simulink model "model"  (R2014a)
settings: Solver=FixedStepDiscrete  StartTime=0.0  StopTime=10  RelTol=1e-3
values from neighbouring files (symbols this model uses):
  BufLen = 4*Fs    [init_model.m]
  delay_fp1 = ceil(delay_qrs-fpdl-fpdi-fpdd)    [init_model.m]
  delay_fp2 = ceil(delay_qrs-fpdl-s)    [init_model.m]
  delay_noise = ceil(noiseds + noisedl)    [init_model.m]
  Fs = signal.fs    [init_model.m]
  s = round(0.06*Fs)    [init_model.m]
undefined symbols (not defined in the file or in its folder): fpad, fpai, fpal, fpbd, fpbi, fpbl, FrameLen, get, gopalakhermite, HR, JayMeasurePts, noiseal, noiseas, noisebl, noisebs, qrsad, qrsah, qrsai, qrsal, qrsbd, qrsbh, qrsbi, qrsbl, qrsgh, qrsgl, rochahermite1, rochahermite2, stlen
undefined symbols (not defined in the file): L1, L2, L3, L4, newL1, newL2
libraries: simulink x16, neural x14, dspbuff3 x4, dspsigops x2, dspsnks4 x1
(part 1 of 2)
Description:
  | Real-time simulation of ECG ischemia detection
settings Model: Creator=Diego Sogari  LastModifiedBy=Usuario

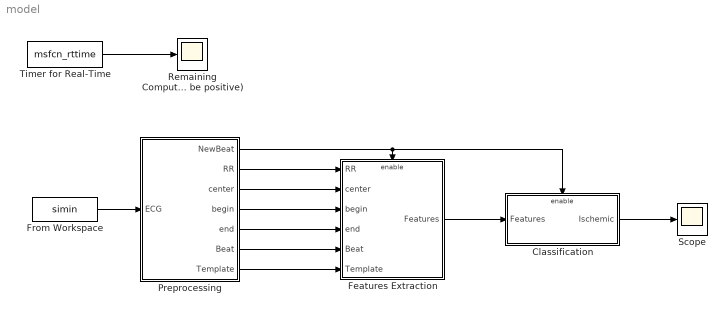
== system model ==
  Classification : Subsystem
  Features Extraction : Subsystem
  From Workspace : FromWorkspace  VariableName=simin  SampleTime=1/Fs  Interpolate=off  OutputAfterFinalValue=Setting to zero
  Preprocessing : Subsystem
  Remaining Computation Time (must be positive) : Scope
      settings: TimeRange=10  YMin=-0.175  YMax=0.025
  Scope : Scope
  Timer for Real-Time : S-Function  FunctionName=msfcn_rttime  Parameters=Fs 1  EnableBusSupport=off
  wires:
  From Workspace/1 -> Preprocessing/1(ECG)
  Preprocessing/5(end) -> Features Extraction/4(end)
  Preprocessing/2(RR) -> Features Extraction/1(RR)
  Preprocessing/3(center) -> Features Extraction/2(center)
  Preprocessing/4(begin) -> Features Extraction/3(begin)
  Classification/1(Ischemic) -> Scope/1
  Timer for Real-Time/1 -> Remaining Computation Time (must be positive)/1
  Preprocessing/1(NewBeat) -> Classification/Enable, Features Extraction/Enable
  Preprocessing/6(Beat) -> Features Extraction/5(Beat)
  Preprocessing/7(Template) -> Features Extraction/6(Template)
  Features Extraction/1(Features) -> Classification/1(Features)

== system model/Classification ==
  Features : Inport
  Enable : EnablePort
  Bus Selector : BusSelector
  Gopalak Networks : Subsystem
  Mohebbi Netowrk : Subsystem
  Rocha Networks : Subsystem
  Vector Concatenate : Concatenate  NumInputs=3
  Ischemic : Outport
  wires:
  Features/1 -> Bus Selector/1
  Bus Selector/3 -> Gopalak Networks/1(Features)  "<signal3>"
  Bus Selector/1 -> Rocha Networks/1(Features)  "<signal1>"
  Bus Selector/2 -> Mohebbi Netowrk/1(Features)  "<signal2>"
  Rocha Networks/1(Ischemic) -> Vector Concatenate/1
  Mohebbi Netowrk/1(Ischemic) -> Vector Concatenate/2
  Gopalak Networks/1(Ischemic) -> Vector Concatenate/3
  Vector Concatenate/1 -> Ischemic/1

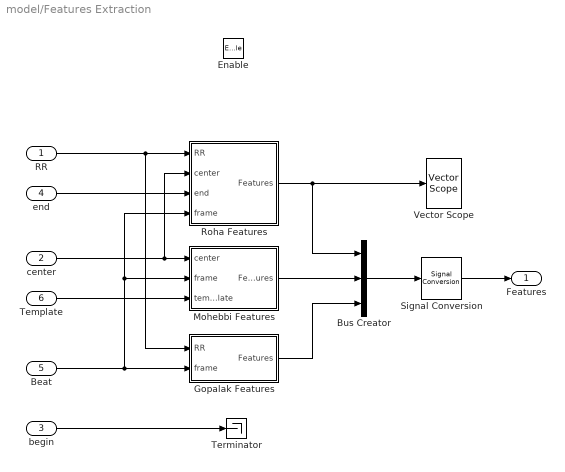
== system model/Features Extraction ==
  RR : Inport
  center : Inport  Port=2
  begin : Inport  Port=3
  end : Inport  Port=4
  Beat : Inport  Port=5
  Template : Inport  Port=6
  Enable : EnablePort
  Bus Creator : BusCreator  Inputs=3
  Gopalak Features : Subsystem
  Mohebbi Features : Subsystem
  Roha Features : Subsystem
  Signal Conversion : SignalConversion
  Terminator : Terminator
  Vector Scope : dspsnks4/Vector Scope  ScopeProperties=on  Domain=Time  HorizSpan=1  DisplayProperties=off  AxisGrid=on  Memory=off  FrameNumber=on  AxisLegend=off  AxisZoom=off  OpenScopeAtSimStart=on  OpenScopeImmediately=off  FigPos=get(0,'defaultfigureposition')  AxisProperties=off  XUnits=Hertz  XRange=[0...Fs/2]  InheritXIncr=on  XIncr=1  XLabel=Time  XLimit=Auto  XMin=0  XMax=1  XStart=0  YUnits=dB  YLabel=Amplitude  LineProperties=off  XAxisParamsVer=6.9
      settings: YMin=-10  YMax=10
  Features : Outport
  wires:
  center/1 -> Roha Features/2(center), Mohebbi Features/1(center)
  RR/1 -> Gopalak Features/1(RR), Roha Features/1(RR)
  end/1 -> Roha Features/3(end)
  Mohebbi Features/1(Features) -> Bus Creator/2
  Roha Features/1(Features) -> Vector Scope/1, Bus Creator/1
  Gopalak Features/1(Features) -> Bus Creator/3
  Beat/1 -> Roha Features/4(frame), Mohebbi Features/2(frame), Gopalak Features/2(frame)
  Template/1 -> Mohebbi Features/3(template)
  begin/1 -> Terminator/1
  Bus Creator/1 -> Signal Conversion/1
  Signal Conversion/1 -> Features/1

== system model/Preprocessing ==
  ECG : Inport
  Filtering : Subsystem
  Subsystem : Subsystem
  NewBeat : Outport
  RR : Outport  Port=2
  center : Outport  Port=3
  begin : Outport  Port=4
  end : Outport  Port=5
  Beat : Outport  Port=6
  Template : Outport  Port=7
  wires:
  ECG/1 -> Filtering/1(Data)
  Filtering/1(QRSsig) -> Subsystem/1(QRSsig)
  Filtering/2(FPsigD) -> Subsystem/2(FPsigD)
  Filtering/3(FPsigM) -> Subsystem/3(FPsigM)
  Filtering/4(Noissig) -> Subsystem/4(Noissig)
  Subsystem/2(RR) -> RR/1
  Subsystem/3(center) -> center/1
  Subsystem/4(begin) -> begin/1
  Subsystem/5(end) -> end/1
  Subsystem/1(NewBeat) -> NewBeat/1
  Subsystem/7(Template) -> Template/1
  Subsystem/6(Beat) -> Beat/1

== system model/Classification/Gopalak Networks ==
  Features : Inport
  Constant : Constant  Value=0  OutDataTypeStr=boolean
  Terminator : Terminator
  Ischemic : Outport
  wires:
  Features/1 -> Terminator/1
  Constant/1 -> Ischemic/1

== system model/Classification/Mohebbi Netowrk ==
  Features : Inport
  Constant : Constant  Value=0  OutDataTypeStr=boolean
  Terminator : Terminator
  Ischemic : Outport
  wires:
  Features/1 -> Terminator/1
  Constant/1 -> Ischemic/1

== system model/Classification/Rocha Networks ==
  Features : Inport
  Compare To Zero : simulink/Logic and Bit Operations/Compare To Zero  relop=>  OutDataTypeStr=boolean
  Feed-Forward Neural Network : Subsystem
      mask help: Feed-Forward Neural Network
      mask Display: e = 0.06;c1 = [120 150 230]/255;c2 = ([120 150 230]+0)/383;c3 = ([120 150 230]+128)/383;patch([0 1 1 0],[0 0 1 1],c1);patch([0 1 1 1-e 1-e 0+e],[0 0 1 1-e 0+e 0+e],c2);patch([0 0 1 1-e 0+e 0+e],[0 1 1 1-e 1-e 0+e],c3);plot([0 1 1 0 0],[0 0 1 1 0]);fprintf('NNET');port_label('input',1,' Input');port_label('output',1,'Output ');
  Ischemic : Outport
  wires:
  Features/1 -> Feed-Forward Neural Network/1(Input)
  Feed-Forward Neural Network/1(Output) -> Compare To Zero/1
  Compare To Zero/1 -> Ischemic/1

== system model/Features Extraction/Gopalak Features ==
  RR : Inport
  frame : Inport  Port=2
  Constant : Constant  Value=gopalakhermite
  Extract Segment : S-Function  FunctionName=msfcn_segmentextractor  Parameters=Fs gopalaksegsize resamplen  EnableBusSupport=off
  Matrix Multiply : Product  Multiplication=Matrix(*)
  segment limits : Subsystem
  Features : Outport
  wires:
  frame/1 -> Extract Segment/1
  RR/1 -> segment limits/1(RR)
  segment limits/1(start) -> Extract Segment/2
  segment limits/2(end) -> Extract Segment/3
  Extract Segment/1 -> Matrix Multiply/2
  Matrix Multiply/1 -> Features/1
  Constant/1 -> Matrix Multiply/1

== system model/Features Extraction/Mohebbi Features ==
  center : Inport
  frame : Inport  Port=2
  template : Inport  Port=3
  Extract ST segment : Subsystem
  Exttract ST difference : Subsystem
  Flsg : Subsystem  mask{trigg=3}
      mask prompts: trigg "Trigger count"
  Sample and Hold : dspsigops/Sample and Hold  trig=Rising edge  initCond=0  latchinput=off
  Sample and Hold1 : dspsigops/Sample and Hold  trig=Rising edge  initCond=0  latchinput=off
  Features : Outport
  wires:
  Sample and Hold/1 -> Extract ST segment/1(frame)
  Exttract ST difference/1(STdiff) -> Features/1
  center/1 -> Extract ST segment/2(center), Exttract ST difference/2(center)
  Flsg/1(flag) -> Sample and Hold1/1, Sample and Hold1/Trigger, Sample and Hold/Trigger
  Sample and Hold1/1 -> Exttract ST difference/Enable
  frame/1 -> Exttract ST difference/3(frame)
  template/1 -> Sample and Hold/1
  Extract ST segment/1(STseg) -> Exttract ST difference/1(refST)

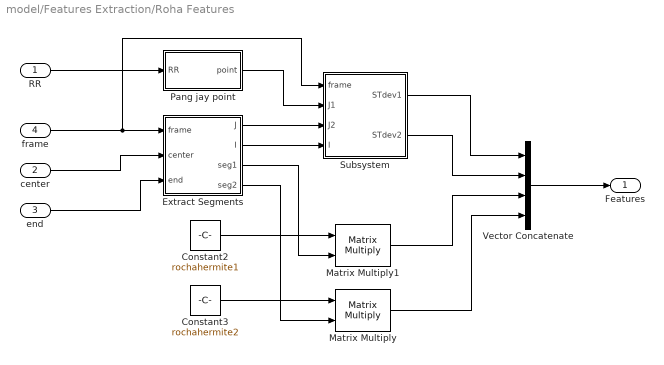
== system model/Features Extraction/Roha Features ==
  RR : Inport
  center : Inport  Port=2
  end : Inport  Port=3
  frame : Inport  Port=4
  Constant2 : Constant  Value=rochahermite1
  Constant3 : Constant  Value=rochahermite2
  Extract Segments : Subsystem
  Matrix Multiply : Product  Multiplication=Matrix(*)
  Matrix Multiply1 : Product  Multiplication=Matrix(*)
  Pang jay point : Subsystem
  Subsystem : Subsystem
  Vector Concatenate : Concatenate  NumInputs=4
  Features : Outport
  wires:
  RR/1 -> Pang jay point/1(RR)
  frame/1 -> Extract Segments/1(frame), Subsystem/1(frame)
  center/1 -> Extract Segments/2(center)
  end/1 -> Extract Segments/3(end)
  Constant2/1 -> Matrix Multiply1/1
  Extract Segments/4(seg2) -> Matrix Multiply/2
  Extract Segments/3(seg1) -> Matrix Multiply1/2
  Matrix Multiply1/1 -> Vector Concatenate/3
  Matrix Multiply/1 -> Vector Concatenate/4
  Vector Concatenate/1 -> Features/1
  Constant3/1 -> Matrix Multiply/1
  Pang jay point/1(point) -> Subsystem/2(J1)
  Extract Segments/1(J) -> Subsystem/3(J2)
  Extract Segments/2(I) -> Subsystem/4(I)
  Subsystem/1(STdev1) -> Vector Concatenate/1
  Subsystem/2(STdev2) -> Vector Concatenate/2

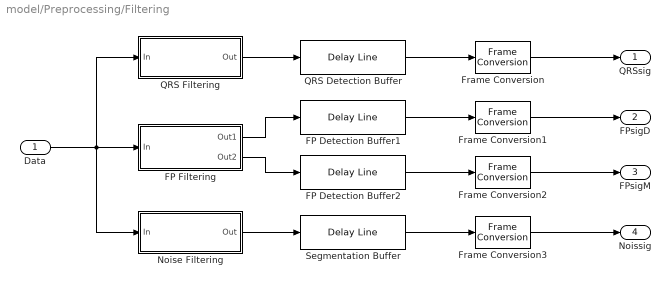
== system model/Preprocessing/Filtering ==
  Data : Inport
  FP Detection Buffer1 : dspbuff3/Delay Line  siz=BufLen  ic=0  directfeed=on  enable_output=off  hold_output=off  TreatMby1Signals=One channel
  FP Detection Buffer2 : dspbuff3/Delay Line  siz=BufLen  ic=0  directfeed=on  enable_output=off  hold_output=off  TreatMby1Signals=One channel
  FP Filtering : Subsystem
  Frame Conversion{,1..3} (4 alike) : FrameConversion  OutFrame=Sample-based
  Noise Filtering : Subsystem
  QRS Detection Buffer : dspbuff3/Delay Line  siz=BufLen  ic=0  directfeed=on  enable_output=off  hold_output=off  TreatMby1Signals=One channel
  QRS Filtering : Subsystem
  Segmentation Buffer : dspbuff3/Delay Line  siz=BufLen  ic=0  directfeed=on  enable_output=off  hold_output=off  TreatMby1Signals=One channel
  QRSsig : Outport
  FPsigD : Outport  Port=2
  FPsigM : Outport  Port=3
  Noissig : Outport  Port=4
  wires:
  Frame Conversion1/1 -> FPsigD/1
  Frame Conversion3/1 -> Noissig/1
  Noise Filtering/1(Out) -> Segmentation Buffer/1
  FP Detection Buffer1/1 -> Frame Conversion1/1
  FP Detection Buffer2/1 -> Frame Conversion2/1
  QRS Filtering/1(Out) -> QRS Detection Buffer/1
  Data/1 -> Noise Filtering/1(In), QRS Filtering/1(In), FP Filtering/1(In)
  FP Filtering/1(Out1) -> FP Detection Buffer1/1
  QRS Detection Buffer/1 -> Frame Conversion/1
  FP Filtering/2(Out2) -> FP Detection Buffer2/1
  Segmentation Buffer/1 -> Frame Conversion3/1
  Frame Conversion2/1 -> FPsigM/1
  Frame Conversion/1 -> QRSsig/1

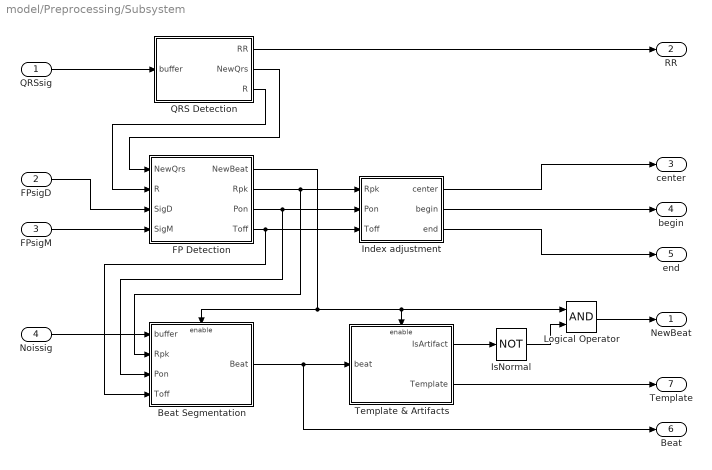
== system model/Preprocessing/Subsystem ==
  QRSsig : Inport
  FPsigD : Inport  Port=2
  FPsigM : Inport  Port=3
  Noissig : Inport  Port=4
  Beat Segmentation : Subsystem
  FP Detection : Subsystem
  Index adjustment : Subsystem
  IsNormal : Logic  Operator=NOT  AllPortsSameDT=off  OutDataTypeStr=boolean
  Logical Operator : Logic  AllPortsSameDT=off  OutDataTypeStr=boolean
  QRS Detection : Subsystem
  Template & Artifacts : Subsystem
  NewBeat : Outport
  RR : Outport  Port=2
  center : Outport  Port=3
  begin : Outport  Port=4
  end : Outport  Port=5
  Beat : Outport  Port=6
  Template : Outport  Port=7
  wires:
  Beat Segmentation/1(Beat) -> Beat/1, Template & Artifacts/1(beat)
  Noissig/1 -> Beat Segmentation/1(buffer)
  FPsigD/1 -> FP Detection/3(SigD)
  QRSsig/1 -> QRS Detection/1(buffer)
  FPsigM/1 -> FP Detection/4(SigM)
  FP Detection/3(Pon) -> Index adjustment/2(Pon), Beat Segmentation/3(Pon)
  QRS Detection/2(NewQrs) -> FP Detection/1(NewQrs)
  QRS Detection/3(R) -> FP Detection/2(R)
  QRS Detection/1(RR) -> RR/1
  FP Detection/2(Rpk) -> Index adjustment/1(Rpk), Beat Segmentation/2(Rpk)
  FP Detection/1(NewBeat) -> Beat Segmentation/Enable, Logical Operator/1, Template & Artifacts/Enable
  Index adjustment/3(end) -> end/1
  FP Detection/4(Toff) -> Index adjustment/3(Toff), Beat Segmentation/4(Toff)
  IsNormal/1 -> Logical Operator/2
  Logical Operator/1 -> NewBeat/1
  Index adjustment/2(begin) -> begin/1
  Template & Artifacts/1(IsArtifact) -> IsNormal/1
  Template & Artifacts/2(Template) -> Template/1
  Index adjustment/1(center) -> center/1

== system model/Classification/Rocha Networks/Feed-Forward Neural Network ==
  Input : Inport  PortDimensions=14  SampleTime=0.004
      mask Display: e = 0.06;c1 = [120 230 180]/255;c2 = ([120 230 180]+0)/(256+128);c3 = ([120 230 180]+128)/(256+128);patch([0 1 1 0],[0 0 1 1],c1);patch([0 1 1 1-e 1-e 0+e],[0 0 1 1-e 0+e 0+e],c2);patch([0 0 1 1-e 0+e 0+e],[0 1 1 1-e 1-e 0+e],c3);plot([0 1 1 0 0],[0 0 1 1 0]);
  Layer 1 : Subsystem
      mask Display: e = 0.06;c1 = [120 150 230]/255;c2 = ([120 150 230]+0)/383;c3 = ([120 150 230]+128)/383;patch([0 1 1 0],[0 0 1 1],c1);patch([0 1 1 1-e 1-e 0+e],[0 0 1 1-e 0+e 0+e],c2);patch([0 0 1 1-e 0+e 0+e],[0 1 1 1-e 1-e 0+e],c3);plot([0 1 1 0 0],[0 0 1 1 0]);
  Layer 2 : Subsystem
      mask Display: e = 0.06;c1 = [120 150 230]/255;c2 = ([120 150 230]+0)/383;c3 = ([120 150 230]+128)/383;patch([0 1 1 0],[0 0 1 1],c1);patch([0 1 1 1-e 1-e 0+e],[0 0 1 1-e 0+e 0+e],c2);patch([0 0 1 1-e 0+e 0+e],[0 1 1 1-e 1-e 0+e],c3);plot([0 1 1 0 0],[0 0 1 1 0]);
  Layer 3 : Subsystem
      mask Display: e = 0.06;c1 = [120 150 230]/255;c2 = ([120 150 230]+0)/383;c3 = ([120 150 230]+128)/383;patch([0 1 1 0],[0 0 1 1],c1);patch([0 1 1 1-e 1-e 0+e],[0 0 1 1-e 0+e 0+e],c2);patch([0 0 1 1-e 0+e 0+e],[0 1 1 1-e 1-e 0+e],c3);plot([0 1 1 0 0],[0 0 1 1 0]);
  Process Input 1 : Subsystem
      mask Display: e = 0.06;c1 = [120 150 230]/255;c2 = ([120 150 230]+0)/383;c3 = ([120 150 230]+128)/383;patch([0 1 1 0],[0 0 1 1],c1);patch([0 1 1 1-e 1-e 0+e],[0 0 1 1-e 0+e 0+e],c2);patch([0 0 1 1-e 0+e 0+e],[0 1 1 1-e 1-e 0+e],c3);plot([0 1 1 0 0],[0 0 1 1 0]);
  Process Output 1 : Subsystem
      mask Display: e = 0.06;c1 = [120 150 230]/255;c2 = ([120 150 230]+0)/383;c3 = ([120 150 230]+128)/383;patch([0 1 1 0],[0 0 1 1],c1);patch([0 1 1 1-e 1-e 0+e],[0 0 1 1-e 0+e 0+e],c2);patch([0 0 1 1-e 0+e 0+e],[0 1 1 1-e 1-e 0+e],c3);plot([0 1 1 0 0],[0 0 1 1 0]);
  Output : Outport  InitialOutput=0
      mask Display: e = 0.06;c1 = [120 230 180]/255;c2 = ([120 230 180]+0)/(256+128);c3 = ([120 230 180]+128)/(256+128);patch([0 1 1 0],[0 0 1 1],c1);patch([0 1 1 1-e 1-e 0+e],[0 0 1 1-e 0+e 0+e],c2);patch([0 0 1 1-e 0+e 0+e],[0 1 1 1-e 1-e 0+e],c3);plot([0 1 1 0 0],[0 0 1 1 0]);
  wires:
  Layer 3/1("a{3}") -> Process Output 1/1(a)
  [feedback2] -> Layer 3/1("a{2} ")
  Layer 2/1("a{2}") -> [feedback2]
  [feedback1] -> Layer 2/1("a{1} ")
  Layer 1/1("a{1}") -> [feedback1]
  Process Input 1/1(p) -> Layer 1/1("p{1}")
  Process Output 1/1(y) -> Output/1
  Input/1 -> Process Input 1/1(x)

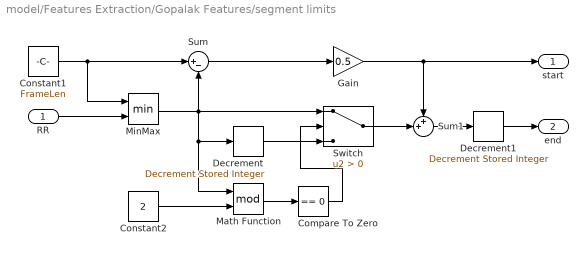
== system model/Features Extraction/Gopalak Features/segment limits ==
  RR : Inport
  Compare To Zero : simulink/Logic and Bit Operations/Compare To Zero  relop===  OutDataTypeStr=boolean
  Constant1 : Constant  Value=FrameLen  OutDataTypeStr=int32
  Constant2 : Constant  Value=2  OutDataTypeStr=int32
  Decrement : simulink/Additional Math & Discrete/Additional Math: Increment - Decrement/Decrement Stored Integer
  Decrement1 : simulink/Additional Math & Discrete/Additional Math: Increment - Decrement/Decrement Stored Integer
  Gain : Gain  Gain=0.5  OutDataTypeStr=int32
  Math Function : Math  Operator=mod  SaturateOnIntegerOverflow=on
  MinMax : MinMax  Inputs=2  OutDataTypeStr=int32
  Sum : Sum  Inputs=|+-
  Sum1 : Sum  Inputs=++|
  Switch : Switch  Criteria=u2 > Threshold
  start : Outport
  end : Outport  Port=2
  wires:
  Gain/1 -> start/1, Sum1/1
  MinMax/1 -> Math Function/1, Decrement/1, Sum/2, Switch/1
  Constant1/1 -> Sum/1, MinMax/1
  Sum/1 -> Gain/1
  RR/1 -> MinMax/2
  Sum1/1 -> Decrement1/1
  Switch/1 -> Sum1/2
  Decrement/1 -> Switch/3
  Constant2/1 -> Math Function/2
  Math Function/1 -> Compare To Zero/1
  Compare To Zero/1 -> Switch/2
  Decrement1/1 -> end/1

== system model/Features Extraction/Mohebbi Features/Extract ST segment ==
  frame : Inport
  center : Inport  Port=2
  Extract Segment : S-Function  FunctionName=msfcn_segmentextractor  Parameters=Fs mohebbisegsize resamplen  EnableBusSupport=off
  STlen : Constant  Value=stlen-1  OutDataTypeStr=int32
  Search jay point : S-Function  FunctionName=msfcn_edgedetector  Parameters=Fs newL1 jaythresh  EnableBusSupport=off
  Smooth and diff : S-Function  FunctionName=msfcn_blockfilter  Parameters=Fs beatfb beatfa beatfd  EnableBusSupport=off
  Sum : Sum  Inputs=|++
  edge limits : Subsystem  mask{searchL1=newL1, searchL2=newL2}
      mask prompts: searchL1 "First search offset (in samples)"; searchL2 "Second search offset (in samples)"
  STseg : Outport
  wires:
  Smooth and diff/1 -> Search jay point/1
  center/1 -> edge limits/1(idx)
  edge limits/2(end) -> Search jay point/3
  edge limits/1(start) -> Search jay point/2
  edge limits/3(def) -> Search jay point/4
  Search jay point/1 -> Sum/1, Extract Segment/2
  STlen/1 -> Sum/2
  Sum/1 -> Extract Segment/3
  Extract Segment/1 -> STseg/1
  frame/1 -> Extract Segment/1, Smooth and diff/1

== system model/Features Extraction/Mohebbi Features/Exttract ST difference ==
  refST : Inport
  center : Inport  Port=2
  frame : Inport  Port=3
  Enable : EnablePort
  Extract ST segment : Subsystem
  Sum : Sum  Inputs=|+-
  STdiff : Outport
  wires:
  frame/1 -> Extract ST segment/1(frame)
  center/1 -> Extract ST segment/2(center)
  Extract ST segment/1(STseg) -> Sum/1
  refST/1 -> Sum/2
  Sum/1 -> STdiff/1

== system model/Features Extraction/Mohebbi Features/Flsg ==
  Beat Count : simulink/Sources/Counter Free-Running  NumBits=16  tsamp=-1
  Compare To Constant : simulink/Logic and Bit Operations/Compare To Constant  relop===  const=trigg  OutDataTypeStr=boolean
  Increment : simulink/Additional Math & Discrete/Additional Math: Increment - Decrement/Increment Stored Integer
  flag : Outport
  wires:
  Increment/1 -> Compare To Constant/1
  Beat Count/1 -> Increment/1
  Compare To Constant/1 -> flag/1

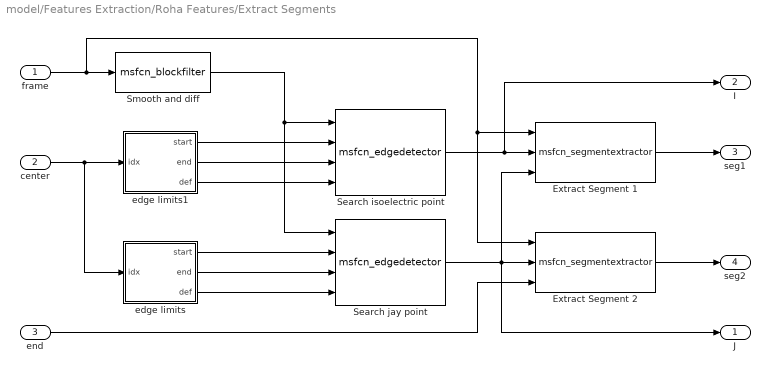
== system model/Features Extraction/Roha Features/Extract Segments ==
  frame : Inport
  center : Inport  Port=2
  end : Inport  Port=3
  Extract Segment 1 : S-Function  FunctionName=msfcn_segmentextractor  Parameters=Fs rochasegsize resamplen  EnableBusSupport=off
  Extract Segment 2 : S-Function  FunctionName=msfcn_segmentextractor  Parameters=Fs rochasegsize resamplen  EnableBusSupport=off
  Search isoelectric point : S-Function  FunctionName=msfcn_edgedetector  Parameters=Fs newL1 jaythresh  EnableBusSupport=off
  Search jay point : S-Function  FunctionName=msfcn_edgedetector  Parameters=Fs newL1 jaythresh  EnableBusSupport=off
  Smooth and diff : S-Function  FunctionName=msfcn_blockfilter  Parameters=Fs beatfb beatfa beatfd  EnableBusSupport=off
  edge limits : Subsystem  mask{searchL1=newL1, searchL2=newL2}
      mask prompts: searchL1 "First search offset (in samples)"; searchL2 "Second search offset (in samples)"
  edge limits1 : Subsystem  mask{searchL1=-newL1, searchL2=-newL2}
      mask prompts: searchL1 "First search offset (in samples)"; searchL2 "Second search offset (in samples)"
  J : Outport
  I : Outport  Port=2
  seg1 : Outport  Port=3
  seg2 : Outport  Port=4
  wires:
  edge limits1/1(start) -> Search isoelectric point/2
  edge limits1/2(end) -> Search isoelectric point/3
  edge limits1/3(def) -> Search isoelectric point/4
  edge limits/3(def) -> Search jay point/4
  edge limits/1(start) -> Search jay point/2
  edge limits/2(end) -> Search jay point/3
  center/1 -> edge limits/1(idx), edge limits1/1(idx)
  frame/1 -> Extract Segment 1/1, Extract Segment 2/1, Smooth and diff/1
  Smooth and diff/1 -> Search jay point/1, Search isoelectric point/1
  Search isoelectric point/1 -> I/1, Extract Segment 1/2
  Search jay point/1 -> J/1, Extract Segment 2/2, Extract Segment 1/3
  end/1 -> Extract Segment 2/3
  Extract Segment 1/1 -> seg1/1
  Extract Segment 2/1 -> seg2/1

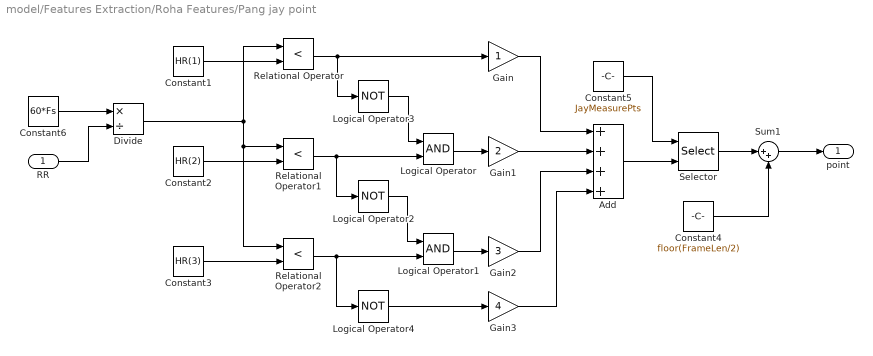
== system model/Features Extraction/Roha Features/Pang jay point ==
  RR : Inport
  Add : Sum  Inputs=++++
  Constant1 : Constant  Value=HR(1)
  Constant2 : Constant  Value=HR(2)
  Constant3 : Constant  Value=HR(3)
  Constant4 : Constant  Value=floor(FrameLen/2)  OutDataTypeStr=int32
  Constant5 : Constant  Value=JayMeasurePts  OutDataTypeStr=int32
  Constant6 : Constant  Value=60*Fs
  Divide : Product  Inputs=*/
  Gain : Gain  OutDataTypeStr=int32
  Gain1 : Gain  Gain=2  OutDataTypeStr=int32
  Gain2 : Gain  Gain=3  OutDataTypeStr=int32
  Gain3 : Gain  Gain=4  OutDataTypeStr=int32
  Logical Operator : Logic  AllPortsSameDT=off  OutDataTypeStr=boolean
  Logical Operator1 : Logic  AllPortsSameDT=off  OutDataTypeStr=boolean
  Logical Operator2 : Logic  Operator=NOT  AllPortsSameDT=off  OutDataTypeStr=boolean
  Logical Operator3 : Logic  Operator=NOT  AllPortsSameDT=off  OutDataTypeStr=boolean
  Logical Operator4 : Logic  Operator=NOT  AllPortsSameDT=off  OutDataTypeStr=boolean
  Relational Operator : RelationalOperator  Operator=<  OutDataTypeStr=boolean
  Relational Operator1 : RelationalOperator  Operator=<  OutDataTypeStr=boolean
  Relational Operator2 : RelationalOperator  Operator=<  OutDataTypeStr=boolean
  Selector : Selector  InputPortWidth=length(JayMeasurePts)  IndexOptions=Index vector (port)  Indices=[1 3]
  Sum1 : Sum  Inputs=|++
  point : Outport
  wires:
  Constant5/1 -> Selector/1
  Add/1 -> Selector/2
  Gain/1 -> Add/1
  Gain1/1 -> Add/2
  Gain2/1 -> Add/3
  Gain3/1 -> Add/4
  Logical Operator1/1 -> Gain2/1
  Logical Operator/1 -> Gain1/1
  Relational Operator/1 -> Logical Operator3/1, Gain/1
  Logical Operator4/1 -> Gain3/1
  Relational Operator2/1 -> Logical Operator4/1, Logical Operator1/2
  Relational Operator1/1 -> Logical Operator/2, Logical Operator2/1
  Logical Operator2/1 -> Logical Operator1/1
  Logical Operator3/1 -> Logical Operator/1
  Constant1/1 -> Relational Operator/2
  Constant2/1 -> Relational Operator1/2
  Constant3/1 -> Relational Operator2/2
  Selector/1 -> Sum1/1
  Constant4/1 -> Sum1/2
  Sum1/1 -> point/1
  Constant6/1 -> Divide/1
  RR/1 -> Divide/2
  Divide/1 -> Relational Operator/1, Relational Operator1/1, Relational Operator2/1

== system model/Features Extraction/Roha Features/Subsystem ==
  frame : Inport
  J1 : Inport  Port=2
  J2 : Inport  Port=3
  I : Inport  Port=4
  Selector : Selector  IndexMode=Zero-based  InputPortWidth=FrameLen  IndexOptions=Index vector (port)  Indices=[1 3]
  Selector1 : Selector  IndexMode=Zero-based  InputPortWidth=FrameLen  IndexOptions=Index vector (port)  Indices=[1 3]
  Selector2 : Selector  IndexMode=Zero-based  InputPortWidth=FrameLen  IndexOptions=Index vector (port)  Indices=[1 3]
  Sum : Sum  Inputs=|+-
  Sum1 : Sum  Inputs=-+|
  STdev1 : Outport
  STdev2 : Outport  Port=2
  wires:
  J2/1 -> Selector/2
  Sum/1 -> STdev1/1
  I/1 -> Selector2/2
  Selector2/1 -> Sum1/1, Sum/2
  Selector1/1 -> Sum/1
  J1/1 -> Selector1/2
  Sum1/1 -> STdev2/1
  Selector/1 -> Sum1/2
  frame/1 -> Selector1/1, Selector2/1, Selector/1

== system model/Preprocessing/Filtering/FP Filtering ==
  In : Inport
  Conversion to int : DataTypeConversion  OutDataTypeStr=int32  LockScale=on
  Delay : Delay  DelayLength=delay_fp1  UseCircularBuffer=on
  Delay1 : Delay  DelayLength=delay_fp2  UseCircularBuffer=on
  Low-pass : DiscreteFilter  Numerator=fpbl  Denominator=fpal  a0EqualsOne=on  StateDataTypeStr=int32  OutDataTypeStr=int32
  Morphological derivative : Subsystem
  Smoothed derivative : Subsystem
  Out1 : Outport
  Out2 : Outport  Port=2
  wires:
  Conversion to int/1 -> Low-pass/1
  In/1 -> Conversion to int/1
  Low-pass/1 -> Smoothed derivative/1(In), Morphological derivative/1(In)
  Delay/1 -> Out1/1
  Delay1/1 -> Out2/1
  Morphological derivative/1(Out) -> Delay1/1
  Smoothed derivative/1(Out) -> Delay/1

== system model/Preprocessing/Filtering/Noise Filtering ==
  In : Inport
  Conversion to double : DataTypeConversion  OutDataTypeStr=double  LockScale=on
  Delay : Delay  DelayLength=delay_noise  UseCircularBuffer=on
  Low-pass : DiscreteFilter  Numerator=noisebl  Denominator=noiseal
  Stop-band : DiscreteFilter  Numerator=noisebs  Denominator=noiseas
  Out : Outport
  wires:
  In/1 -> Conversion to double/1
  Low-pass/1 -> Delay/1
  Stop-band/1 -> Low-pass/1
  Delay/1 -> Out/1
  Conversion to double/1 -> Stop-band/1

== system model/Preprocessing/Filtering/QRS Filtering ==
  In : Inport
  Differentiator : DiscreteFilter  Numerator=qrsbd  Denominator=qrsad  a0EqualsOne=on  StateDataTypeStr=int16  OutDataTypeStr=int16
  High-pass : Subsystem
  Low-pass : Subsystem
  Moving-average : DiscreteFilter  Numerator=qrsbi  Denominator=qrsai  a0EqualsOne=on  StateDataTypeStr=int32  OutDataTypeStr=int32
  Squaring : Subsystem
  Out : Outport
  wires:
  Moving-average/1 -> Out/1
  In/1 -> Low-pass/1(In)
  Low-pass/1(Out) -> High-pass/1(In)
  High-pass/1(Out) -> Differentiator/1
  Differentiator/1 -> Squaring/1(In)
  Squaring/1(Out) -> Moving-average/1

== system model/Preprocessing/Subsystem/Beat Segmentation ==
  buffer : Inport
  Rpk : Inport  Port=2
  Pon : Inport  Port=3
  Toff : Inport  Port=4
  Enable : EnablePort
  S-Function : S-Function  FunctionName=msfcn_baselinefit  Parameters=Fs 5  EnableBusSupport=off
  S-Function2 : S-Function  FunctionName=msfcn_beatframer  Parameters=Fs FrameLen  EnableBusSupport=off
  Beat : Outport
  wires:
  Toff/1 -> S-Function2/4, S-Function/3
  Pon/1 -> S-Function2/3, S-Function/2
  S-Function/1 -> S-Function2/5
  Rpk/1 -> S-Function2/2
  S-Function2/1 -> Beat/1
  buffer/1 -> S-Function2/1, S-Function/1

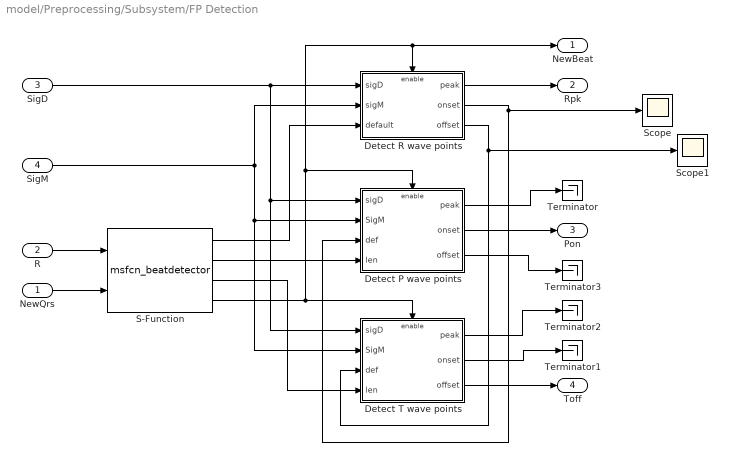
== system model/Preprocessing/Subsystem/FP Detection ==
  NewQrs : Inport
  R : Inport  Port=2
  SigD : Inport  Port=3
  SigM : Inport  Port=4
  Detect P wave points : Subsystem
  Detect R wave points : Subsystem
  Detect T wave points : Subsystem
  S-Function : S-Function  FunctionName=msfcn_beatdetector  Parameters=Fs  EnableBusSupport=off
  Scope : Scope
      settings: SaveName=ScopeData3
  Scope1 : Scope
      settings: SaveName=ScopeData4
  Terminator{,1..3} (4 alike) : Terminator
  NewBeat : Outport
  Rpk : Outport  Port=2
  Pon : Outport  Port=3
  Toff : Outport  Port=4
  wires:
  NewQrs/1 -> S-Function/2
  R/1 -> S-Function/1
  SigD/1 -> Detect T wave points/1(sigD), Detect P wave points/1(sigD), Detect R wave points/1(sigD)
  SigM/1 -> Detect T wave points/2(SigM), Detect P wave points/2(SigM), Detect R wave points/2(sigM)
  Detect R wave points/1(peak) -> Rpk/1
  S-Function/1 -> Detect R wave points/3(default)
  Detect T wave points/2(onset) -> Terminator1/1
  Detect T wave points/3(offset) -> Toff/1
  Detect T wave points/1(peak) -> Terminator2/1
  S-Function/4 -> Detect T wave points/Enable, Detect R wave points/Enable, NewBeat/1, Detect P wave points/Enable
  S-Function/2 -> Detect P wave points/4(len)
  S-Function/3 -> Detect T wave points/4(len)
  Detect R wave points/2(onset) -> Detect P wave points/3(def), Scope/1
  Detect R wave points/3(offset) -> Scope1/1, Detect T wave points/3(def)
  Detect P wave points/1(peak) -> Terminator/1
  Detect P wave points/2(onset) -> Pon/1
  Detect P wave points/3(offset) -> Terminator3/1

== system model/Preprocessing/Subsystem/Index adjustment ==
  Rpk : Inport
  Pon : Inport  Port=2
  Toff : Inport  Port=3
  Constant : Constant  Value=floor(FrameLen/2)  OutDataTypeStr=int32
  Sum : Sum  Inputs=|-+
  Sum1 : Sum  Inputs=++|
  Sum2 : Sum  Inputs=+-|
  Sum3 : Sum  Inputs=-+|
  center : Outport
  begin : Outport  Port=2
  end : Outport  Port=3
  wires:
  Sum/1 -> Sum2/2
  Sum3/1 -> Sum1/2
  Sum2/1 -> begin/1
  Constant/1 -> center/1, Sum1/1, Sum2/1
  Sum1/1 -> end/1
  Pon/1 -> Sum/1
  Rpk/1 -> Sum/2, Sum3/1
  Toff/1 -> Sum3/2

== system model/Preprocessing/Subsystem/QRS Detection ==
  buffer : Inport
  Detect Peak : Subsystem
  Evaluate Peaks : Subsystem
  Evaluate QRS : Subsystem
  Training : Subsystem  mask{TP=2}
      mask prompts: TP "Training Period (in seconds)"
  RR : Outport
  NewQrs : Outport  Port=2
  R : Outport  Port=3
  wires:
  Training/1(Flag) -> Evaluate Peaks/4(training)
  Evaluate Peaks/1(peakIdx) -> Evaluate QRS/2(peak), R/1
  Evaluate Peaks/2(thresh) -> Evaluate QRS/3(thresh)
  Evaluate Peaks/3(validated) -> Evaluate QRS/4(validated)
  Evaluate Peaks/4(detected) -> Evaluate QRS/5(detected)
  Evaluate QRS/1(NewQrs) -> NewQrs/1
  Evaluate QRS/2(sbackIdx) -> Evaluate Peaks/5(sbackIdx)
  Evaluate QRS/3(rrMean) -> RR/1
  Detect Peak/1(peakIdx) -> Evaluate Peaks/2(currIdx)
  Detect Peak/2(detected) -> Evaluate Peaks/3(newPeak)
  Detect Peak/3(rising) -> Evaluate QRS/6(rising)
  buffer/1 -> Evaluate Peaks/1(signal), Evaluate QRS/1(buffer), Detect Peak/1(buffer)

== system model/Preprocessing/Subsystem/Template & Artifacts ==
  beat : Inport
  Enable : EnablePort
  Template Builder : S-Function  FunctionName=msfcn_templatebuilder  Parameters=Fs TempCount  EnableBusSupport=off
  Terminator : Terminator
  IsArtifact : Outport
  Template : Outport  Port=2
  wires:
  beat/1 -> Template Builder/1
  Template Builder/1 -> Template/1
  Template Builder/3 -> IsArtifact/1
  Template Builder/2 -> Terminator/1

== system model/Classification/Rocha Networks/Feed-Forward Neural Network/Layer 1 ==
  "p{1}" : Inport  PortDimensions=14  SampleTime=0.004
      mask Display: e = 0.06;c1 = [120 230 180]/255;c2 = ([120 230 180]+0)/(256+128);c3 = ([120 230 180]+128)/(256+128);patch([0 1 1 0],[0 0 1 1],c1);patch([0 1 1 1-e 1-e 0+e],[0 0 1 1-e 0+e 0+e],c2);patch([0 0 1 1-e 0+e 0+e],[0 1 1 1-e 1-e 0+e],c3);plot([0 1 1 0 0],[0 0 1 1 0]);
  Delays 1 : Subsystem
      mask Display: e = 0.06;c1 = [120 150 230]/255;c2 = ([120 150 230]+0)/383;c3 = ([120 150 230]+128)/383;patch([0 1 1 0],[0 0 1 1],c1);patch([0 1 1 1-e 1-e 0+e],[0 0 1 1-e 0+e 0+e],c2);patch([0 0 1 1-e 0+e 0+e],[0 1 1 1-e 1-e 0+e],c3);plot([0 1 1 0 0],[0 0 1 1 0]);disp('0');
  "IW{1,1}" : Subsystem
      mask Display: e = 0.06;c1 = [120 150 230]/255;c2 = ([120 150 230]+0)/383;c3 = ([120 150 230]+128)/383;patch([0 1 1 0],[0 0 1 1],c1);patch([0 1 1 1-e 1-e 0+e],[0 0 1 1-e 0+e 0+e],c2);patch([0 0 1 1-e 0+e 0+e],[0 1 1 1-e 1-e 0+e],c3);plot([0 1 1 0 0],[0 0 1 1 0]);disp('W');
  "b{1}" : Constant  Value=[-1.9119333728239882;-0.12991537511162193;-107.3533300736394;-0.99878670506974421;4.3327736636178216]
      mask Display: e = 0.06;c1 = [120 150 230]/255;c2 = ([120 150 230]+0)/383;c3 = ([120 150 230]+128)/383;patch([0 1 1 0],[0 0 1 1],c1);patch([0 1 1 1-e 1-e 0+e],[0 0 1 1-e 0+e 0+e],c2);patch([0 0 1 1-e 0+e 0+e],[0 1 1 1-e 1-e 0+e],c3);plot([0 1 1 0 0],[0 0 1 1 0]);disp('b');
  netsum : Sum  Inputs=2  SaturateOnIntegerOverflow=on  InputSameDT=on  OutDataTypeStr=Inherit: Same as first input
      mask Display: e = 0.06;c1 = [120 150 230]/255;c2 = ([120 150 230]+0)/383;c3 = ([120 150 230]+128)/383;patch([0 1 1 0],[0 0 1 1],c1);patch([0 1 1 1-e 1-e 0+e],[0 0 1 1-e 0+e 0+e],c2);patch([0 0 1 1-e 0+e 0+e],[0 1 1 1-e 1-e 0+e],c3);plot([0 1 1 0 0],[0 0 1 1 0]);disp('+');
  tansig : neural/Transfer Functions/tansig
  "a{1}" : Outport  InitialOutput=[0;0;0;0;0]
      mask Display: e = 0.06;c1 = [120 230 180]/255;c2 = ([120 230 180]+0)/(256+128);c3 = ([120 230 180]+128)/(256+128);patch([0 1 1 0],[0 0 1 1],c1);patch([0 1 1 1-e 1-e 0+e],[0 0 1 1-e 0+e 0+e],c2);patch([0 0 1 1-e 0+e 0+e],[0 1 1 1-e 1-e 0+e],c3);plot([0 1 1 0 0],[0 0 1 1 0]);
  wires:
  tansig/1 -> "a{1}"/1
  netsum/1 -> tansig/1
  "b{1}"/1 -> netsum/2
  "IW{1,1}"/1("iz{1,1}") -> netsum/1
  Delays 1/1("pd{1,1}") -> "IW{1,1}"/1("pd{1,1}")
  "p{1}"/1 -> Delays 1/1("p{1}")

== system model/Classification/Rocha Networks/Feed-Forward Neural Network/Layer 2 ==
  "a{1} " : Inport  PortDimensions=5  SampleTime=0.004
      mask Display: e = 0.06;c1 = [120 230 180]/255;c2 = ([120 230 180]+0)/(256+128);c3 = ([120 230 180]+128)/(256+128);patch([0 1 1 0],[0 0 1 1],c1);patch([0 1 1 1-e 1-e 0+e],[0 0 1 1-e 0+e 0+e],c2);patch([0 0 1 1-e 0+e 0+e],[0 1 1 1-e 1-e 0+e],c3);plot([0 1 1 0 0],[0 0 1 1 0]);
  Delays 1 : Subsystem
      mask Display: e = 0.06;c1 = [120 150 230]/255;c2 = ([120 150 230]+0)/383;c3 = ([120 150 230]+128)/383;patch([0 1 1 0],[0 0 1 1],c1);patch([0 1 1 1-e 1-e 0+e],[0 0 1 1-e 0+e 0+e],c2);patch([0 0 1 1-e 0+e 0+e],[0 1 1 1-e 1-e 0+e],c3);plot([0 1 1 0 0],[0 0 1 1 0]);disp('0');
  "LW{2,1}" : Subsystem
      mask Display: e = 0.06;c1 = [120 150 230]/255;c2 = ([120 150 230]+0)/383;c3 = ([120 150 230]+128)/383;patch([0 1 1 0],[0 0 1 1],c1);patch([0 1 1 1-e 1-e 0+e],[0 0 1 1-e 0+e 0+e],c2);patch([0 0 1 1-e 0+e 0+e],[0 1 1 1-e 1-e 0+e],c3);plot([0 1 1 0 0],[0 0 1 1 0]);disp('W');
  "b{2}" : Constant  Value=[-188.1608776590252;189.58415083552043;256.10242057871824]
      mask Display: e = 0.06;c1 = [120 150 230]/255;c2 = ([120 150 230]+0)/383;c3 = ([120 150 230]+128)/383;patch([0 1 1 0],[0 0 1 1],c1);patch([0 1 1 1-e 1-e 0+e],[0 0 1 1-e 0+e 0+e],c2);patch([0 0 1 1-e 0+e 0+e],[0 1 1 1-e 1-e 0+e],c3);plot([0 1 1 0 0],[0 0 1 1 0]);disp('b');
  netsum : Sum  Inputs=2  SaturateOnIntegerOverflow=on  InputSameDT=on  OutDataTypeStr=Inherit: Same as first input
      mask Display: e = 0.06;c1 = [120 150 230]/255;c2 = ([120 150 230]+0)/383;c3 = ([120 150 230]+128)/383;patch([0 1 1 0],[0 0 1 1],c1);patch([0 1 1 1-e 1-e 0+e],[0 0 1 1-e 0+e 0+e],c2);patch([0 0 1 1-e 0+e 0+e],[0 1 1 1-e 1-e 0+e],c3);plot([0 1 1 0 0],[0 0 1 1 0]);disp('+');
  tansig : neural/Transfer Functions/tansig
  "a{2}" : Outport  InitialOutput=[0;0;0]
      mask Display: e = 0.06;c1 = [120 230 180]/255;c2 = ([120 230 180]+0)/(256+128);c3 = ([120 230 180]+128)/(256+128);patch([0 1 1 0],[0 0 1 1],c1);patch([0 1 1 1-e 1-e 0+e],[0 0 1 1-e 0+e 0+e],c2);patch([0 0 1 1-e 0+e 0+e],[0 1 1 1-e 1-e 0+e],c3);plot([0 1 1 0 0],[0 0 1 1 0]);
  wires:
  tansig/1 -> "a{2}"/1
  netsum/1 -> tansig/1
  "b{2}"/1 -> netsum/2
  "LW{2,1}"/1("lz{2,1}") -> netsum/1
  Delays 1/1("pd{2,1}") -> "LW{2,1}"/1("ad{2,1}")
  "a{1} "/1 -> Delays 1/1("p{2}")

== system model/Classification/Rocha Networks/Feed-Forward Neural Network/Layer 3 ==
  "a{2} " : Inport  PortDimensions=3  SampleTime=0.004
      mask Display: e = 0.06;c1 = [120 230 180]/255;c2 = ([120 230 180]+0)/(256+128);c3 = ([120 230 180]+128)/(256+128);patch([0 1 1 0],[0 0 1 1],c1);patch([0 1 1 1-e 1-e 0+e],[0 0 1 1-e 0+e 0+e],c2);patch([0 0 1 1-e 0+e 0+e],[0 1 1 1-e 1-e 0+e],c3);plot([0 1 1 0 0],[0 0 1 1 0]);
  Delays 1 : Subsystem
      mask Display: e = 0.06;c1 = [120 150 230]/255;c2 = ([120 150 230]+0)/383;c3 = ([120 150 230]+128)/383;patch([0 1 1 0],[0 0 1 1],c1);patch([0 1 1 1-e 1-e 0+e],[0 0 1 1-e 0+e 0+e],c2);patch([0 0 1 1-e 0+e 0+e],[0 1 1 1-e 1-e 0+e],c3);plot([0 1 1 0 0],[0 0 1 1 0]);disp('0');
  "LW{3,2}" : Subsystem
      mask Display: e = 0.06;c1 = [120 150 230]/255;c2 = ([120 150 230]+0)/383;c3 = ([120 150 230]+128)/383;patch([0 1 1 0],[0 0 1 1],c1);patch([0 1 1 1-e 1-e 0+e],[0 0 1 1-e 0+e 0+e],c2);patch([0 0 1 1-e 0+e 0+e],[0 1 1 1-e 1-e 0+e],c3);plot([0 1 1 0 0],[0 0 1 1 0]);disp('W');
  "b{3}" : Constant  Value=0.09892635476406407
      mask Display: e = 0.06;c1 = [120 150 230]/255;c2 = ([120 150 230]+0)/383;c3 = ([120 150 230]+128)/383;patch([0 1 1 0],[0 0 1 1],c1);patch([0 1 1 1-e 1-e 0+e],[0 0 1 1-e 0+e 0+e],c2);patch([0 0 1 1-e 0+e 0+e],[0 1 1 1-e 1-e 0+e],c3);plot([0 1 1 0 0],[0 0 1 1 0]);disp('b');
  netsum : Sum  Inputs=2  SaturateOnIntegerOverflow=on  InputSameDT=on  OutDataTypeStr=Inherit: Same as first input
      mask Display: e = 0.06;c1 = [120 150 230]/255;c2 = ([120 150 230]+0)/383;c3 = ([120 150 230]+128)/383;patch([0 1 1 0],[0 0 1 1],c1);patch([0 1 1 1-e 1-e 0+e],[0 0 1 1-e 0+e 0+e],c2);patch([0 0 1 1-e 0+e 0+e],[0 1 1 1-e 1-e 0+e],c3);plot([0 1 1 0 0],[0 0 1 1 0]);disp('+');
  purelin : neural/Transfer Functions/purelin
  "a{3}" : Outport  InitialOutput=0
      mask Display: e = 0.06;c1 = [120 230 180]/255;c2 = ([120 230 180]+0)/(256+128);c3 = ([120 230 180]+128)/(256+128);patch([0 1 1 0],[0 0 1 1],c1);patch([0 1 1 1-e 1-e 0+e],[0 0 1 1-e 0+e 0+e],c2);patch([0 0 1 1-e 0+e 0+e],[0 1 1 1-e 1-e 0+e],c3);plot([0 1 1 0 0],[0 0 1 1 0]);
  wires:
  purelin/1 -> "a{3}"/1
  netsum/1 -> purelin/1
  "b{3}"/1 -> netsum/2
  "LW{3,2}"/1("lz{3,2}") -> netsum/1
  Delays 1/1("pd{3,2}") -> "LW{3,2}"/1("ad{3,2}")
  "a{2} "/1 -> Delays 1/1("p{3}")

== system model/Classification/Rocha Networks/Feed-Forward Neural Network/Process Input 1 ==
  x : Inport  PortDimensions=14  SampleTime=0.004
      mask Display: e = 0.06;c1 = [120 230 180]/255;c2 = ([120 230 180]+0)/(256+128);c3 = ([120 230 180]+128)/(256+128);patch([0 1 1 0],[0 0 1 1],c1);patch([0 1 1 1-e 1-e 0+e],[0 0 1 1-e 0+e 0+e],c2);patch([0 0 1 1-e 0+e 0+e],[0 1 1 1-e 1-e 0+e],c3);plot([0 1 1 0 0],[0 0 1 1 0]);
  mapminmax : neural/Processing Functions/mapminmax  xmin=[-311.95112329633895;-292.40146140899401;-1186.4293275097496;-1314.0533037940345;-664.93979314836145;-970.35176038342036;-579.98063961252933;-594.92967360047635;-1272.7169783909762;-607.77830002314397;-677.46672042264652;-526.36596099663518;-439.62494918242936;-345.71867672987571]  xmax=[246.19998549233929;209.32187097750821;2294.8529464241992;1277.0392703148427;1150.3315978648886;830.08466715444126;934.1877535123707;698.62692673270749;949.7930377783274;687.52144976723059;766.10413219824602;397.46109931387247;535.22971554300727;366.69691187555753]  ymin=-1  ymax=1
  p : Outport  PortDimensions=14  SampleTime=0.004
      mask Display: e = 0.06;c1 = [120 230 180]/255;c2 = ([120 230 180]+0)/(256+128);c3 = ([120 230 180]+128)/(256+128);patch([0 1 1 0],[0 0 1 1],c1);patch([0 1 1 1-e 1-e 0+e],[0 0 1 1-e 0+e 0+e],c2);patch([0 0 1 1-e 0+e 0+e],[0 1 1 1-e 1-e 0+e],c3);plot([0 1 1 0 0],[0 0 1 1 0]);
  wires:
  mapminmax/1 -> p/1
  x/1 -> mapminmax/1

== system model/Classification/Rocha Networks/Feed-Forward Neural Network/Process Output 1 ==
  a : Inport  PortDimensions=1  SampleTime=0.004
      mask Display: e = 0.06;c1 = [120 230 180]/255;c2 = ([120 230 180]+0)/(256+128);c3 = ([120 230 180]+128)/(256+128);patch([0 1 1 0],[0 0 1 1],c1);patch([0 1 1 1-e 1-e 0+e],[0 0 1 1-e 0+e 0+e],c2);patch([0 0 1 1-e 0+e 0+e],[0 1 1 1-e 1-e 0+e],c3);plot([0 1 1 0 0],[0 0 1 1 0]);
  mapminmax_reverse : neural/Processing Functions/mapminmax_reverse  xmin=-1  xmax=1  ymin=-1  ymax=1
  y : Outport  PortDimensions=1  SampleTime=0.004
      mask Display: e = 0.06;c1 = [120 230 180]/255;c2 = ([120 230 180]+0)/(256+128);c3 = ([120 230 180]+128)/(256+128);patch([0 1 1 0],[0 0 1 1],c1);patch([0 1 1 1-e 1-e 0+e],[0 0 1 1-e 0+e 0+e],c2);patch([0 0 1 1-e 0+e 0+e],[0 1 1 1-e 1-e 0+e],c3);plot([0 1 1 0 0],[0 0 1 1 0]);
  wires:
  mapminmax_reverse/1 -> y/1
  a/1 -> mapminmax_reverse/1

== system model/Features Extraction/Mohebbi Features/Extract ST segment/edge limits ==
  idx : Inport
  Constant1 : Constant  Value=searchL1  OutDataTypeStr=int32
  Constant2 : Constant  Value=searchL2  OutDataTypeStr=int32
  Sum : Sum  Inputs=++|
  Sum1 : Sum  Inputs=|++
  start : Outport
  end : Outport  Port=2
  def : Outport  Port=3
  wires:
  Sum1/1 -> start/1
  Sum/1 -> end/1
  Constant2/1 -> Sum/2
  Constant1/1 -> Sum1/1
  idx/1 -> Sum1/2, Sum/1, def/1

== system model/Features Extraction/Mohebbi Features/Exttract ST difference/Extract ST segment ==
  frame : Inport
  center : Inport  Port=2
  Extract Segment : S-Function  FunctionName=msfcn_segmentextractor  Parameters=Fs mohebbisegsize resamplen  EnableBusSupport=off
  STlen : Constant  Value=stlen-1  OutDataTypeStr=int32
  Search jay point : S-Function  FunctionName=msfcn_edgedetector  Parameters=Fs newL1 jaythresh  EnableBusSupport=off
  Smooth and diff : S-Function  FunctionName=msfcn_blockfilter  Parameters=Fs beatfb beatfa beatfd  EnableBusSupport=off
  Sum : Sum  Inputs=|++
  edge limits : Subsystem  mask{searchL1=newL1, searchL2=newL2}
      mask prompts: searchL1 "First search offset (in samples)"; searchL2 "Second search offset (in samples)"
  STseg : Outport
  wires:
  Smooth and diff/1 -> Search jay point/1
  center/1 -> edge limits/1(idx)
  edge limits/2(end) -> Search jay point/3
  edge limits/1(start) -> Search jay point/2
  edge limits/3(def) -> Search jay point/4
  Search jay point/1 -> Sum/1, Extract Segment/2
  STlen/1 -> Sum/2
  Sum/1 -> Extract Segment/3
  Extract Segment/1 -> STseg/1
  frame/1 -> Extract Segment/1, Smooth and diff/1

== system model/Features Extraction/Roha Features/Extract Segments/edge limits ==
  idx : Inport
  Constant1 : Constant  Value=searchL1  OutDataTypeStr=int32
  Constant2 : Constant  Value=searchL2  OutDataTypeStr=int32
  Sum : Sum  Inputs=++|
  Sum1 : Sum  Inputs=|++
  start : Outport
  end : Outport  Port=2
  def : Outport  Port=3
  wires:
  idx/1 -> def/1, Sum/1, Sum1/2
  Constant1/1 -> Sum1/1
  Constant2/1 -> Sum/2
  Sum/1 -> end/1
  Sum1/1 -> start/1

== system model/Features Extraction/Roha Features/Extract Segments/edge limits1 ==
  idx : Inport
  Constant1 : Constant  Value=searchL1  OutDataTypeStr=int32
  Constant2 : Constant  Value=searchL2  OutDataTypeStr=int32
  Sum : Sum  Inputs=++|
  Sum1 : Sum  Inputs=|++
  start : Outport
  end : Outport  Port=2
  def : Outport  Port=3
  wires:
  Sum1/1 -> start/1
  Sum/1 -> end/1
  Constant2/1 -> Sum/2
  Constant1/1 -> Sum1/1
  idx/1 -> Sum1/2, Sum/1, def/1

== system model/Preprocessing/Filtering/FP Filtering/Morphological derivative ==
  In : Inport
  Add : Sum  Inputs=++-  AccumDataTypeStr=int32  OutDataTypeStr=int32
  Delay2 : Delay  DelayLength=s  UseCircularBuffer=on
  Gain : Gain  Gain=2  OutDataTypeStr=int32
  S-Function : S-Function  FunctionName=msfcn_rminmax  Parameters=Fs fpeds false  EnableBusSupport=off
  S-Function1 : S-Function  FunctionName=msfcn_rminmax  Parameters=Fs fpeds true  EnableBusSupport=off
  Out : Outport
  wires:
  S-Function/1 -> Add/1
  S-Function1/1 -> Add/2
  In/1 -> S-Function/1, S-Function1/1, Delay2/1
  Delay2/1 -> Gain/1
  Gain/1 -> Add/3
  Add/1 -> Out/1

== system model/Preprocessing/Filtering/FP Filtering/Smoothed derivative ==
  In : Inport
  Differentiator : DiscreteFilter  Numerator=fpbd  Denominator=fpad  a0EqualsOne=on  OutDataTypeStr=int32
  Moving-average : DiscreteFilter  Numerator=fpbi  Denominator=fpai  a0EqualsOne=on  OutDataTypeStr=int32
  Out : Outport
  wires:
  Moving-average/1 -> Differentiator/1
  Differentiator/1 -> Out/1
  In/1 -> Moving-average/1

== system model/Preprocessing/Filtering/QRS Filtering/High-pass ==
  In : Inport
  Constant2 : Constant  Value=qrsgh  OutDataTypeStr=int32
  Discrete Filter : DiscreteFilter  Numerator=qrsbh  Denominator=qrsah  a0EqualsOne=on  StateDataTypeStr=int32  OutDataTypeStr=int32
  Divide2 : Product  Inputs=*/  OutDataTypeStr=int16
  Out : Outport
  wires:
  In/1 -> Discrete Filter/1
  Discrete Filter/1 -> Divide2/1
  Constant2/1 -> Divide2/2
  Divide2/1 -> Out/1

== system model/Preprocessing/Filtering/QRS Filtering/Low-pass ==
  In : Inport
  Constant1 : Constant  Value=qrsgl  OutDataTypeStr=int32
  Discrete Filter : DiscreteFilter  Numerator=qrsbl  Denominator=qrsal  a0EqualsOne=on  StateDataTypeStr=int32  OutDataTypeStr=int32
  Divide1 : Product  Inputs=*/  OutDataTypeStr=int16
  Out : Outport
  wires:
  Constant1/1 -> Divide1/2
  In/1 -> Discrete Filter/1
  Divide1/1 -> Out/1
  Discrete Filter/1 -> Divide1/1

== system model/Preprocessing/Filtering/QRS Filtering/Squaring ==
  In : Inport
  Constant : Constant  Value=2^3  OutDataTypeStr=double
  Divide : Product  Inputs=*/  OutDataTypeStr=double
  Math Function : Math  Operator=square  OutDataTypeStr=double  SaturateOnIntegerOverflow=on
  Saturation : Saturate  UpperLimit=2^15-1  LowerLimit=0  OutDataTypeStr=int16
      settings: LockScale=on
  Out : Outport
  wires:
  Math Function/1 -> Divide/1
  Divide/1 -> Saturation/1
  Saturation/1 -> Out/1
  In/1 -> Math Function/1
  Constant/1 -> Divide/2

== system model/Preprocessing/Subsystem/FP Detection/Detect P wave points ==
  sigD : Inport
  SigM : Inport  Port=2
  def : Inport  Port=3
  len : Inport  Port=4
  Enable : EnablePort
  Search onset and offset : Subsystem
  Search peak : S-Function  FunctionName=msfcn_searchpeak  Parameters=Fs  EnableBusSupport=off
  peak limits : Subsystem  mask{searchL1=-1, searchL2Mult=-0.375}
      mask prompts: searchL1 "First search offset (in samples)"; searchL2Mult "Second search offset multiplier"
  peak : Outport
  onset : Outport  Port=2
  offset : Outport  Port=3
  wires:
  SigM/1 -> Search peak/2, Search onset and offset/1(buffM)
  sigD/1 -> Search peak/1
  def/1 -> peak limits/1(idx)
  Search onset and offset/1(onset) -> onset/1
  len/1 -> peak limits/2(len)
  peak limits/1(start) -> Search peak/3
  Search peak/1 -> peak/1, Search onset and offset/2(peak)
  Search onset and offset/2(offset) -> offset/1
  peak limits/2(end) -> Search peak/4
  peak limits/3(def) -> Search peak/5

== system model/Preprocessing/Subsystem/FP Detection/Detect R wave points ==
  sigD : Inport
  sigM : Inport  Port=2
  default : Inport  Port=3
  Enable : EnablePort
  Search onset and offset : Subsystem
  Search peak : S-Function  FunctionName=msfcn_searchpeak  Parameters=Fs  EnableBusSupport=off
  peak limits : Subsystem  mask{searchL1=-L1, searchL2=L1}
      mask prompts: searchL1 "First search offset (in samples)"; searchL2 "Second search offset (in samples)"
  peak : Outport
  onset : Outport  Port=2
  offset : Outport  Port=3
  wires:
  Search onset and offset/2(offset) -> offset/1
  peak limits/2(end) -> Search peak/4
  peak limits/1(start) -> Search peak/3
  default/1 -> peak limits/1(idx)
  Search onset and offset/1(onset) -> onset/1
  peak limits/3(def) -> Search peak/5
  sigD/1 -> Search peak/1
  sigM/1 -> Search peak/2, Search onset and offset/1(buffM)
  Search peak/1 -> peak/1, Search onset and offset/2(peak)

== system model/Preprocessing/Subsystem/FP Detection/Detect T wave points ==
  sigD : Inport
  SigM : Inport  Port=2
  def : Inport  Port=3
  len : Inport  Port=4
  Enable : EnablePort
  Search onset and offset : Subsystem
  Search peak : S-Function  FunctionName=msfcn_searchpeak  Parameters=Fs  EnableBusSupport=off
  peak limits : Subsystem  mask{searchL1=1, searchL2Mult=0.5}
      mask prompts: searchL1 "First search offset (in samples)"; searchL2Mult "Second search offset multiplier"
  peak : Outport
  onset : Outport  Port=2
  offset : Outport  Port=3
  wires:
  peak limits/3(def) -> Search peak/5
  peak limits/2(end) -> Search peak/4
  Search onset and offset/2(offset) -> offset/1
  Search peak/1 -> Search onset and offset/2(peak), peak/1
  peak limits/1(start) -> Search peak/3
  len/1 -> peak limits/2(len)
  Search onset and offset/1(onset) -> onset/1
  def/1 -> peak limits/1(idx)
  sigD/1 -> Search peak/1
  SigM/1 -> Search onset and offset/1(buffM), Search peak/2

== system model/Preprocessing/Subsystem/QRS Detection/Detect Peak ==
  buffer : Inport
  Constant : Constant  Value=BufLen
  Peak Detector : S-Function  FunctionName=msfcn_peakdetector  Parameters=Fs  EnableBusSupport=off
  Selector : Selector  InputPortWidth=BufLen  IndexOptions=Index vector (port)  Indices=[1 3]
  peakIdx : Outport
  detected : Outport  Port=2
  rising : Outport  Port=3
  wires:
  Constant/1 -> Selector/2
  Selector/1 -> Peak Detector/1
  Peak Detector/3 -> rising/1
  Peak Detector/1 -> peakIdx/1
  Peak Detector/2 -> detected/1
  buffer/1 -> Selector/1

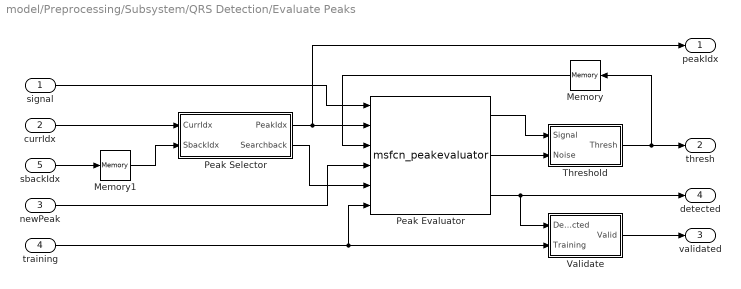
== system model/Preprocessing/Subsystem/QRS Detection/Evaluate Peaks ==
  signal : Inport
  currIdx : Inport  Port=2
  newPeak : Inport  Port=3
  training : Inport  Port=4
  sbackIdx : Inport  Port=5
  Memory : Memory  LinearizeMemory=on
  Memory1 : Memory  LinearizeMemory=on
  Peak Evaluator : S-Function  FunctionName=msfcn_peakevaluator  Parameters=Fs 8  EnableBusSupport=off
  Peak Selector : Subsystem
  Threshold : Subsystem
  Validate : Subsystem
  peakIdx : Outport
  thresh : Outport  Port=2
  validated : Outport  Port=3
  detected : Outport  Port=4
  wires:
  Peak Evaluator/2 -> Threshold/2(Noise)
  Threshold/1(Thresh) -> thresh/1, Memory/1
  Peak Evaluator/3 -> Validate/1(Detected), detected/1
  Peak Selector/2(Searchback) -> Peak Evaluator/5
  Peak Selector/1(PeakIdx) -> Peak Evaluator/2, peakIdx/1
  Peak Evaluator/1 -> Threshold/1(Signal)
  Validate/1(Valid) -> validated/1
  currIdx/1 -> Peak Selector/1(CurrIdx)
  sbackIdx/1 -> Memory1/1
  Memory/1 -> Peak Evaluator/3
  Memory1/1 -> Peak Selector/2(SbackIdx)
  training/1 -> Validate/2(Training), Peak Evaluator/6
  newPeak/1 -> Peak Evaluator/4
  signal/1 -> Peak Evaluator/1

== system model/Preprocessing/Subsystem/QRS Detection/Evaluate QRS ==
  buffer : Inport
  peak : Inport  Port=2
  thresh : Inport  Port=3
  validated : Inport  Port=4
  detected : Inport  Port=5
  rising : Inport  Port=6
  QRS Evaluator : S-Function  FunctionName=msfcn_qrsevaluator  Parameters=Fs  EnableBusSupport=off
  RR Measurer : S-Function  FunctionName=msfcn_rrmeasurer  Parameters=Fs  EnableBusSupport=off
  Search Back : S-Function  FunctionName=msfcn_searchback  Parameters=Fs  EnableBusSupport=off
  NewQrs : Outport
  sbackIdx : Outport  Port=2
  rrMean : Outport  Port=3
  wires:
  QRS Evaluator/1 -> NewQrs/1, RR Measurer/3, Search Back/7
  detected/1 -> RR Measurer/2
  RR Measurer/2 -> Search Back/5
  validated/1 -> QRS Evaluator/3
  rising/1 -> Search Back/6
  thresh/1 -> Search Back/3
  RR Measurer/1 -> rrMean/1, Search Back/4
  Search Back/1 -> sbackIdx/1
  peak/1 -> Search Back/2, QRS Evaluator/2, RR Measurer/1
  buffer/1 -> Search Back/1, QRS Evaluator/1

== system model/Preprocessing/Subsystem/QRS Detection/Training ==
  Clock : Clock
  Compare To Zero : simulink/Logic and Bit Operations/Compare To Zero  relop=<  OutDataTypeStr=boolean
  Sum : Sum  Inputs=|+-
  Training Period : Constant  Value=TP  OutDataTypeStr=int32
  Flag : Outport
  wires:
  Compare To Zero/1 -> Flag/1
  Training Period/1 -> Sum/2
  Sum/1 -> Compare To Zero/1
  Clock/1 -> Sum/1
